simulink model "work4"  (R2026a)
settings: Solver=ode45  StopTime=5  RelTol=1e-8  AbsTol=1e-10
settings Model: Creator=m  LastModifiedBy=m

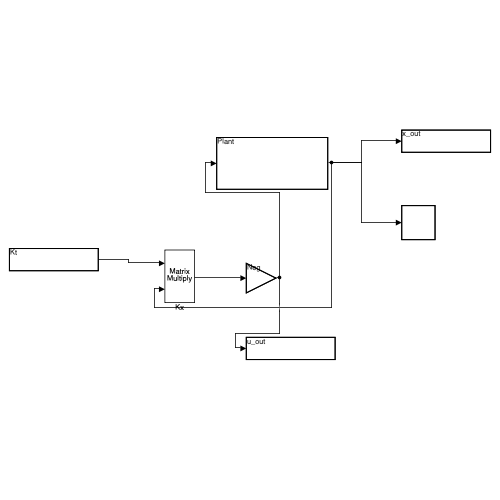
[thumbnail: Simulink's stored preview of the top-level diagram]
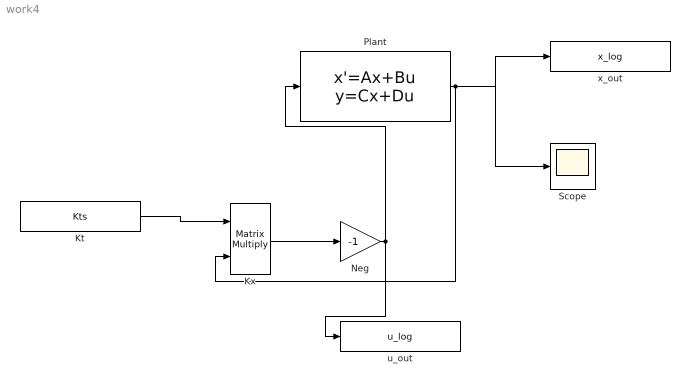
== system work4 ==
  Kt : FromWorkspace  VariableName=Kts  OutputAfterFinalValue=Holding final value
  Kx : Product  Multiplication=Matrix(*)
  Neg : Gain  Gain=-1
  Plant : StateSpace  A=[0 1;-6 -5]  B=[0;1]  C=[1 0;0 1]  D=[0;0]  InitialCondition=[1;0]
  Scope : Scope
  u_out : ToWorkspace  VariableName=u_log  SaveFormat=Timeseries  SampleTime=-1
  x_out : ToWorkspace  VariableName=x_log  SaveFormat=Timeseries  SampleTime=-1
  wires:
  Kt/1 -> Kx/1
  Plant/1 -> Kx/2, x_out/1, Scope/1
  Kx/1 -> Neg/1
  Neg/1 -> Plant/1, u_out/1
